simulink model "verify_HeatPump_basic_mdl"  (R2016b)
settings: Solver=ode45  StartTime=0.0  StopTime=3600  MaxStep=100  RelTol=1e-3  EnableMultiTasking=on
libraries: carnot x5
settings Model: Creator=drhf  LastModifiedBy=srrt
settings DataIOCC: LimitDataPoints=on  SaveFormat=Array  SignalLoggingSaveFormat=ModelDataLogs
settings OptimizationCC: ExpressionDepthLimit=2147483647  LifeSpan=inf
settings DebuggingCC: UnderspecifiedInitializationDetection=Classic  MergeDetectMultiDrivingBlocksExec=none  SolverPrmCheckMsg=warning  FcnCallInpInsideContextMsg=warning  StateNameClashWarn=warning  SFUnexpectedBacktrackingDiag=warning  SFNoUnconditionalDefaultTransitionDiag=warning  SFExecutionAtInitializationDiag=none
settings HardwareCC: ProdBitPerPointer=32  ProdBitPerSizeT=32  ProdBitPerPtrDiffT=32  ProdLargestAtomicFloat=None  ProdIntDivRoundTo=Undefined  ProdEndianess=Unspecified  ProdWordSize=32  ProdHWDeviceType=32-bit Generic
settings ModelReferenceCC: PropagateSignalLabelsOutOfModel=off
settings GRTTargetCC: TargetLangStandard=C89/C90 (ANSI)  GeneratePreprocessorConditionals=Disable all  CombineOutputUpdateFcns=off  GRTInterface=on
settings ConfigComp: CovMetricSettings=dw  CovHtmlReporting=on  CovSaveCumulativeToWorkspaceVar=on  CovSaveSingleToWorkspaceVar=on  CovExternalEMLEnable=off

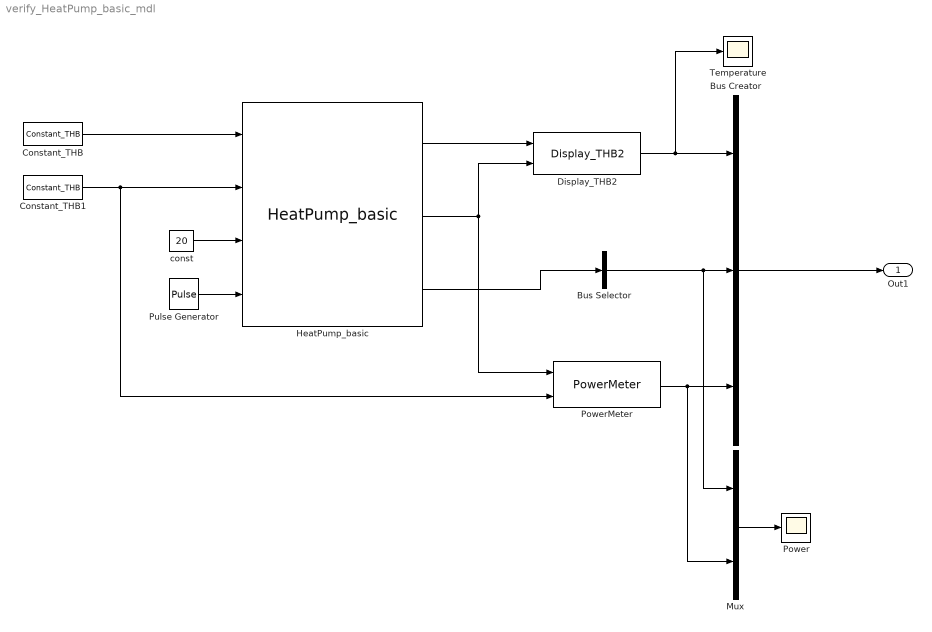
== system verify_HeatPump_basic_mdl ==
  Bus Creator : BusCreator  Inputs=3
  Bus Selector : BusSelector  OutputSignals=Pelec,Qdot_cold,Qdot_hot  OutputAsBus=on
  Constant_THB : carnot/Source/Simple/Constant_THB  t=5  mdot=2000/3600  p=1e5  mID=No Pressure Drop  fluid=Water  mix=0  mix2=0  mix3=0  dia=0.02  hgt=0
  Constant_THB1 : carnot/Source/Simple/Constant_THB  t=40  mdot=2000/3600  p=1e5  mID=No Pressure Drop  fluid=Water  mix=0  mix2=0  mix3=0  dia=0.02  hgt=0
  Display_THB2 : carnot/Outputs/Display_THB2  t=on  m=off  p=off  id=off  mix=off  d=off
  HeatPump_basic : carnot/Basic/Thermal_Models/HeatPump_basic  K="[300 -60 1250  -6.67   60   -5.13e-5   306.7   -115 12225]"  caph=5*4182  capc=5*4182  UA=1
  Mux : Mux  Inputs=2
  Power : Scope
  PowerMeter : carnot/Control/PowerMeter
  Pulse Generator : DiscretePulseGenerator  PulseType=Time based  Period=10*60  PulseWidth=50
  Temperature : Scope
  const : Constant  Value=20
  Out1 : Outport
  wires:
  Bus Creator/1 -> Out1/1
  Pulse Generator/1 -> HeatPump_basic/4
  const/1 -> HeatPump_basic/3
  Constant_THB/1 -> HeatPump_basic/1
  Constant_THB1/1 -> HeatPump_basic/2, PowerMeter/2
  HeatPump_basic/1 -> Display_THB2/1
  HeatPump_basic/2 -> PowerMeter/1, Display_THB2/2
  HeatPump_basic/3 -> Bus Selector/1
  Display_THB2/1 -> Temperature/1, Bus Creator/1
  Bus Selector/1 -> Mux/1, Bus Creator/2
  PowerMeter/1 -> Mux/2, Bus Creator/3
  Mux/1 -> Power/1
